simulink model "LinearizedModel60LQRPosition"  (R2020b)
settings: Solver=VariableStepAuto  StartTime=0.0  StopTime=10.0  RelTol=1e-3
values from neighbouring files (symbols this model uses):
  A = sys.a    [LinMod60rpmForLqr.m]    (also in SymbolicEvaluationXhat.m = double(A))
  B = sys.b    [LinMod60rpmForLqr.m]    (also in OtterFunction_EKF.m = 1.08; OtterFunction_lqr.m = 1.08)
  Cfull = sys.c    [LinMod60rpmForLqr.m]
  Dfull = sys.d    [LinMod60rpmForLqr.m]
  N = inv(Dcgain)    [LinMod60rpmForLqr.m]
undefined symbols (not defined in the file or in its folder): F
settings Model: Creator=rapha  LastModifiedBy=rapha

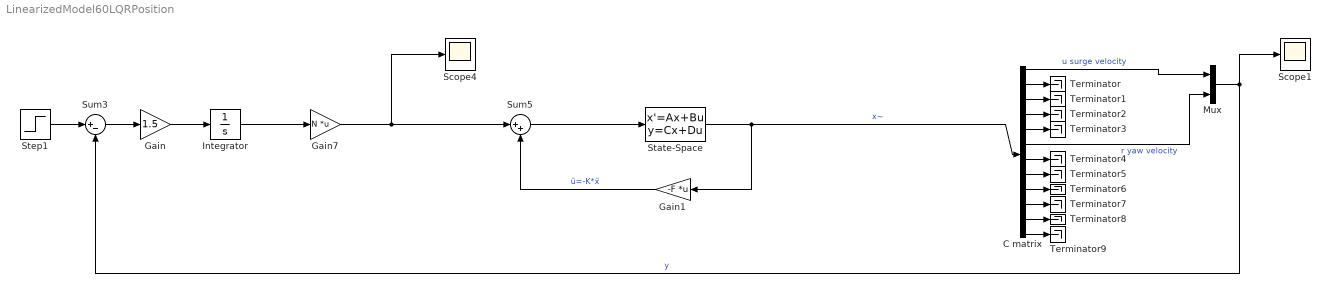
== system LinearizedModel60LQRPosition ==
  C matrix : Demux  Outputs=12
  Gain : Gain  Gain=1.5
  Gain1 : Gain  Gain=-F  Multiplication=Matrix(K*u)
  Gain7 : Gain  Gain=N  Multiplication=Matrix(K*u)
  Integrator : Integrator
  Mux : Mux  Inputs=2
  Scope1 : Scope
  Scope4 : Scope
  State-Space : StateSpace  A=A  B=B  C=Cfull  D=Dfull  InitialCondition=[0 0 0 0 0 0 0 0 0 0 0 0]
  Step1 : Step  After=[1.05 4]  SampleTime=0
  Sum3 : Sum  Inputs=|+-
  Sum5 : Sum  Inputs=|++
  Terminator{,1..9} (10 alike) : Terminator
  wires:
  State-Space/1 -> Gain1/1, C matrix/1  "x~"
  Gain1/1 -> Sum5/2  "ũ=-K*x̃"
  C matrix/6 -> Mux/2  "r yaw velocity"
  C matrix/10 -> Terminator7/1
  C matrix/3 -> Terminator1/1
  C matrix/4 -> Terminator2/1
  C matrix/1 -> Mux/1  "u surge velocity"
  C matrix/12 -> Terminator9/1
  C matrix/8 -> Terminator5/1
  C matrix/7 -> Terminator4/1
  C matrix/11 -> Terminator8/1
  C matrix/2 -> Terminator/1
  C matrix/5 -> Terminator3/1
  C matrix/9 -> Terminator6/1
  Gain7/1 -> Scope4/1, Sum5/1
  Step1/1 -> Sum3/1
  Sum5/1 -> State-Space/1
  Mux/1 -> Scope1/1, Sum3/2  "y"
  Integrator/1 -> Gain7/1
  Sum3/1 -> Gain/1
  Gain/1 -> Integrator/1
